simulink model "estimator2"  (Simulink 8.1)
settings: Solver=ode45  StartTime=0.0  StopTime=10.0  RelTol=1e-3
values from neighbouring files (symbols this model uses):
  A = [-1.5 -0.5;-0.5 -1.0]    [optimiser_setup.m]
  B = [2; -1]    [optimiser_setup.m]
  C = [1 0]    [optimiser_setup.m]
  K = -K    [optimiser_setup.m]
  x1 = (A-B*K)*x0    [optimiser_setup.m]
undefined symbols (not defined in the file or in its folder): L, x1h
libraries: Is_equal_scalar x1, goal x1
settings Model: Creator=dejanira  LastModifiedBy=dejanira
settings DataIOCC: SignalLoggingSaveFormat=Dataset
settings OptimizationCC: ExpressionDepthLimit=128
settings DebuggingCC: FcnCallInpInsideContextMsg=EnableAllAsError
settings GRTTargetCC: CombineOutputUpdateFcns=on  GRTInterface=off

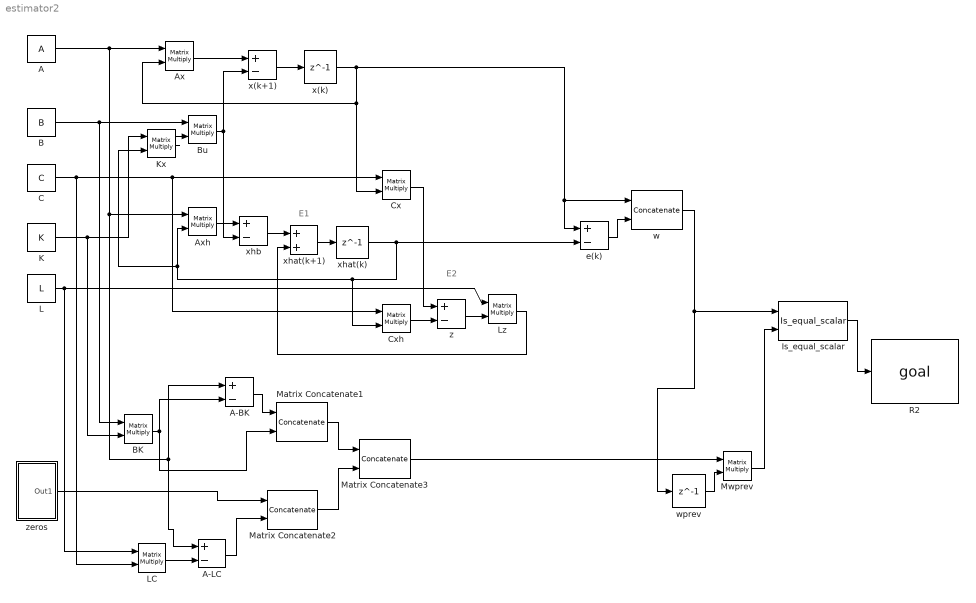
== system estimator2 ==
  note: E1
  note: E2
  A : Constant  Value=A  VectorParams1D=off
  A-BK : Sum  Inputs=+-
  A-LC : Sum  Inputs=+-
  Ax : Product  Multiplication=Matrix(*)
  Axh : Product  Multiplication=Matrix(*)
  B : Constant  Value=B  VectorParams1D=off
  BK : Product  Multiplication=Matrix(*)
  Bu : Product  Multiplication=Matrix(*)
  C : Constant  Value=C  VectorParams1D=off
  Cx : Product  Multiplication=Matrix(*)
  Cxh : Product  Multiplication=Matrix(*)
  Is_equal_scalar : Is_equal_scalar/Is_equal_scalar  SystemSampleTime=-1
  K : Constant  Value=K  VectorParams1D=off
  Kx : Product  Multiplication=Matrix(*)
  L : Constant  Value=L  VectorParams1D=off
  LC : Product  Multiplication=Matrix(*)
  Lz : Product  Multiplication=Matrix(*)
  Matrix Concatenate1 : Concatenate  Mode=Multidimensional array  ConcatenateDimension=2
  Matrix Concatenate2 : Concatenate  Mode=Multidimensional array  ConcatenateDimension=2
  Matrix Concatenate3 : Concatenate  Mode=Multidimensional array
  Mwprev : Product  Multiplication=Matrix(*)
  R2 : goal/goal  SystemSampleTime=-1
  e(k) : Sum  Inputs=+-
  w : Concatenate  Mode=Multidimensional array
  wprev : Delay  DelayLength=1  InitialCondition=x1  SampleTime=0.1
  x(k) : Delay  DelayLength=1  InitialCondition=x1  SampleTime=0.1
  x(k+1) : Sum  Inputs=+-
  xhat(k) : Delay  DelayLength=1  InitialCondition=x1h
  xhat(k+1) : Sum
  xhb : Sum  Inputs=+-
  z : Sum  Inputs=+-
  zeros : Subsystem  mask(m0){}
  wires:
  A/1 -> Ax/1, Axh/1, A-LC/1, A-BK/1
  xhat(k)/1 -> e(k)/2, Cxh/2, Kx/2, Axh/2
  xhat(k+1)/1 -> xhat(k)/1
  z/1 -> Lz/2
  x(k)/1 -> Cx/2, Ax/2, w/1, e(k)/1
  L/1 -> Lz/1, LC/1
  Is_equal_scalar/1 -> R2/1
  Lz/1 -> xhat(k+1)/2
  Matrix Concatenate3/1 -> Mwprev/1
  wprev/1 -> Mwprev/2
  Mwprev/1 -> Is_equal_scalar/2
  e(k)/1 -> w/2
  Matrix Concatenate1/1 -> Matrix Concatenate3/1
  Matrix Concatenate2/1 -> Matrix Concatenate3/2
  w/1 -> wprev/1, Is_equal_scalar/1
  A-LC/1 -> Matrix Concatenate2/2
  C/1 -> Cx/1, Cxh/1, LC/2
  Cx/1 -> z/1
  Cxh/1 -> z/2
  Ax/1 -> x(k+1)/1
  x(k+1)/1 -> x(k)/1
  B/1 -> BK/1, Bu/1
  Bu/1 -> xhb/2, x(k+1)/2
  xhb/1 -> xhat(k+1)/1
  Axh/1 -> xhb/1
  BK/1 -> A-BK/2, Matrix Concatenate1/2
  Kx/1 -> Bu/2
  K/1 -> BK/2, Kx/1
  A-BK/1 -> Matrix Concatenate1/1
  zeros/1(Out1) -> Matrix Concatenate2/1
  LC/1 -> A-LC/2

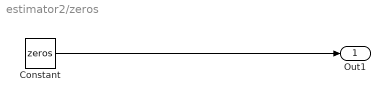
== system estimator2/zeros ==
  Constant : Constant  Value=zeros  VectorParams1D=off
  Out1 : Outport
  wires:
  Constant/1 -> Out1/1
